simulink model "bh_2dof_NP_compare_lagr_vs_sm"  (R2017a)
settings: Solver=ode45  StartTime=0.0  StopTime=60  FixedStep=0.001  RelTol=1e-7  EnableMultiTasking=on
values from neighbouring files (symbols this model uses):
  theta1_0 = 0    [bh_SIMPARAMS_for_2dof_NP_Control_sim.m]
  theta1_dot_0 = 0    [bh_SIMPARAMS_for_2dof_NP_Control_sim.m]
  theta4_0 = 0    [bh_SIMPARAMS_for_2dof_NP_Control_sim.m]
  theta4_dot_0 = 0    [bh_SIMPARAMS_for_2dof_NP_Control_sim.m]
undefined symbols (not defined in the file or in its folder): b1_damp, b4_damp, g, Hz, L1x, L1y, L1z, mass1, mass4, Rturn, sigbuilder_block, X, Y, Z
libraries: simulink_extras x14, sm_lib x13, nesl_utility x9
settings Model: Creator=bhorton  LastModifiedBy=bhorton
settings SolverCC: ZeroCrossAlgorithm=Adaptive
settings OptimizationCC: LifeSpan=inf
settings DebuggingCC: SFUnexpectedBacktrackingDiag=warning  SFNoUnconditionalDefaultTransitionDiag=warning  SFExecutionAtInitializationDiag=none
settings GRTTargetCC: TargetLangStandard=C89/C90 (ANSI)
settings ConfigComp: CovMetricSettings=dw  CovHtmlReporting=on  CovSaveCumulativeToWorkspaceVar=on  CovSaveSingleToWorkspaceVar=on  CovExternalEMLEnable=off
settings SimscapeCC: SimscapeLogDataHistory=10000  SelectedTab=Simscape Multibody
settings ExplorerConfigSet: InternalSimMechanicsExplorerSettings="<ExplorerConfiguration><canonicalview>default</canonicalview><AnimationSetting><BasePlaybackSpeed>1.0</BasePlaybackSpeed><PlaybackSpeedFactor>1.0</PlaybackSpeedFactor></AnimationSetting><TilePanel><TileInfo><Tiles Columns=\"1\" Count=\"1\" Rows=\"1\"><Column Left=\"2\" Weight=\"1\"/><Column Left=\"820\" Weight=\"0.5006\"/><Row Top=\"2\" Weight=\"1\"/><Row Top=\"545\" Weight=\"0.5005\"/><Tile Height=\"1\" Width=\"1\" X=\"0\" Y=\"0\"/></Tiles></TileInfo><SceneInfo><SceneViewer><BGColor><R>0.60000002384185791</R><G>0.60000002384185791</G><B>0.60000002384185791</B></BGColor><Camera><DoPerspective>off</DoPerspective><Position><X>0.48444555295969882</X><Y>-0.15819555793399154</Y><Z>0.39694556248721286</Z></Position><Center><X>0.024999979464140232</X><Y>0.30125001556156705</Y><Z>-0.062500011008345735</Z></Center><Up><X>-0.40824829046386307</X><Y>0.40824829046386307</Y><Z>0.81649658092772615</Z></Up><ViewLimDist>1</ViewLimDist><YLim>0.27384785473346712</YLim><XLim>0.4148743716842227</XLim></Camera></SceneViewer></SceneInfo></TilePanel><MechEditorPanel><Cameras/><GfxPanelCameraMap/></MechEditorPanel></ExplorerConfiguration>"

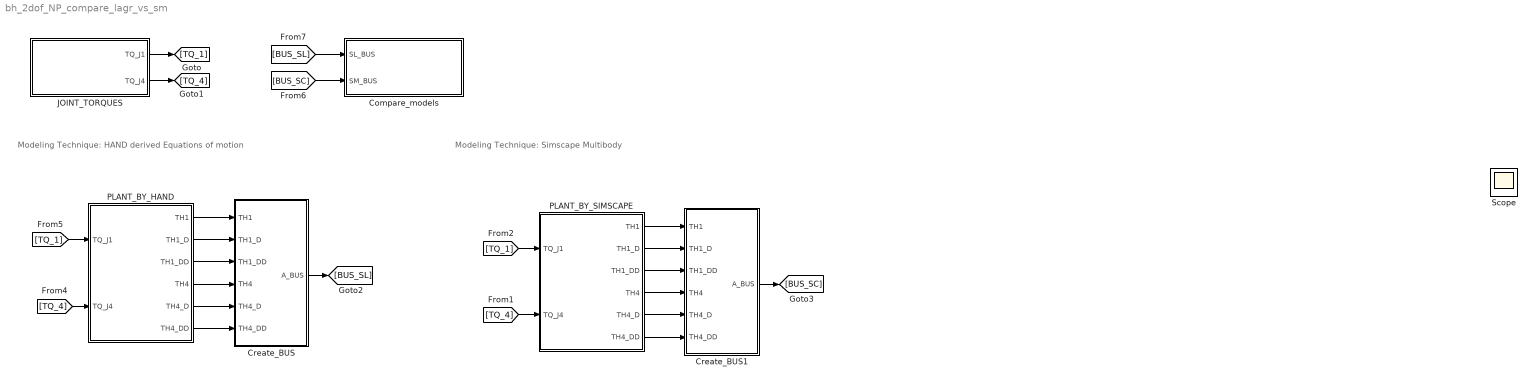
== system bh_2dof_NP_compare_lagr_vs_sm ==
  note: Modeling Technique: HAND derived Equations of motion
  note: Modeling Technique: Simscape Multibody
  Compare_models : Subsystem
  Create_BUS : Subsystem
  Create_BUS1 : Subsystem
  JOINT_TORQUES : Subsystem  Tag=STV Subsys  LoadFcn=sigbuilder_block('load');  StartFcn=sigbuilder_block('start');  StopFcn=sigbuilder_block('stop');  ClipboardFcn=sigbuilder_block('clipboard');  mask(Sigbuilder block){tuvar=[0:10]}
      mask help: Simulink:masks:SigbuilderBlock_MD
      mask init:
      | if ~strcmp(get_param(bdroot(gcbh),'SimulationStatus'),'stopped') tuvar = sigbuilder_block('maskInit'); end
      settings: CopyFcn=sigbuilder_block('copy');  DeleteFcn=sigbuilder_block('delete');  ModelCloseFcn=sigbuilder_block('modelClose');  PreSaveFcn=sigbuilder_block('preSave');  PauseFcn=sigbuilder_block('pause');  ContinueFcn=sigbuilder_block('continue');  NameChangeFcn=sigbuilder_block('namechange');  OpenFcn=sigbuilder_block('open',[6 30 1428 681.75 ]);  CloseFcn=sigbuilder_block('close');
      mask Display: plot(0, 0, 100, 100,[2, 2, 32, 32, 2], [68, 8, 8, 68, 68],[32, 2], [38, 38], [32, 19, 2],[53, 60, 44], [32, 17, 17, 2],[16, 16, 31, 31]);txt = getActiveGroup(gcbh);text(2, 100, txt,'verticalAlignment', 'top');
  PLANT_BY_HAND : Subsystem
  PLANT_BY_SIMSCAPE : Subsystem
  Scope : Scope
  wires:
  JOINT_TORQUES/1(TQ_J1) -> [TQ_1]
  JOINT_TORQUES/2(TQ_J4) -> [TQ_4]
  PLANT_BY_HAND/1(TH1) -> Create_BUS/1(TH1)
  PLANT_BY_HAND/2(TH1_D) -> Create_BUS/2(TH1_D)
  PLANT_BY_HAND/3(TH1_DD) -> Create_BUS/3(TH1_DD)
  PLANT_BY_HAND/4(TH4) -> Create_BUS/4(TH4)
  PLANT_BY_HAND/5(TH4_D) -> Create_BUS/5(TH4_D)
  PLANT_BY_HAND/6(TH4_DD) -> Create_BUS/6(TH4_DD)
  Create_BUS/1(A_BUS) -> [BUS_SL]
  PLANT_BY_SIMSCAPE/1(TH1) -> Create_BUS1/1(TH1)
  PLANT_BY_SIMSCAPE/2(TH1_D) -> Create_BUS1/2(TH1_D)
  PLANT_BY_SIMSCAPE/3(TH1_DD) -> Create_BUS1/3(TH1_DD)
  PLANT_BY_SIMSCAPE/4(TH4) -> Create_BUS1/4(TH4)
  PLANT_BY_SIMSCAPE/5(TH4_D) -> Create_BUS1/5(TH4_D)
  PLANT_BY_SIMSCAPE/6(TH4_DD) -> Create_BUS1/6(TH4_DD)
  Create_BUS1/1(A_BUS) -> [BUS_SC]
  [TQ_1] -> PLANT_BY_HAND/1("TQ_J1 ")
  [TQ_4] -> PLANT_BY_HAND/2(TQ_J4)
  [TQ_1] -> PLANT_BY_SIMSCAPE/1("TQ_J1 ")
  [TQ_4] -> PLANT_BY_SIMSCAPE/2(TQ_J4)
  [BUS_SL] -> Compare_models/1(SL_BUS)
  [BUS_SC] -> Compare_models/2(SM_BUS)

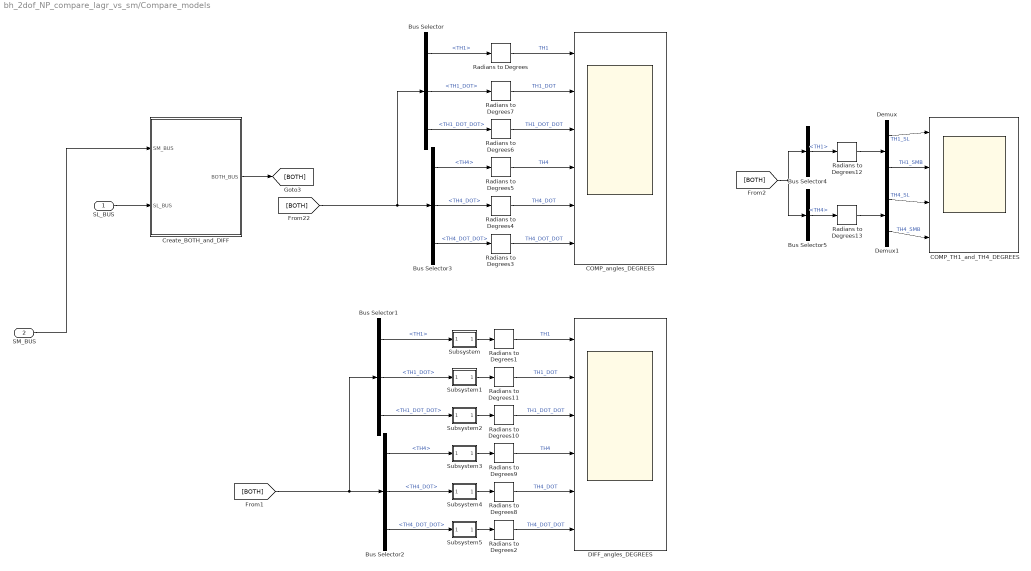
== system bh_2dof_NP_compare_lagr_vs_sm/Compare_models ==
  SL_BUS : Inport
  SM_BUS : Inport  Port=2
  Bus Selector : BusSelector  OutputSignals=TH1,TH1_DOT,TH1_DOT_DOT
  Bus Selector1 : BusSelector  OutputSignals=TH1,TH1_DOT,TH1_DOT_DOT
  Bus Selector2 : BusSelector  OutputSignals=TH4,TH4_DOT,TH4_DOT_DOT
  Bus Selector3 : BusSelector  OutputSignals=TH4,TH4_DOT,TH4_DOT_DOT
  Bus Selector4 : BusSelector  OutputSignals=TH1
  Bus Selector5 : BusSelector  OutputSignals=TH4
  COMP_TH1_and_TH4_DEGREES : Scope  NumInputPorts=4
  COMP_angles_DEGREES : Scope  NumInputPorts=6
  Create_BOTH_and_DIFF : Subsystem
  DIFF_angles_DEGREES : Scope  NumInputPorts=6
  Demux : Demux  Outputs=2
  Demux1 : Demux  Outputs=2
  Radians to Degrees{,1..13} (14 alike) : simulink_extras/Transformations/Radians to Degrees
  Subsystem : Subsystem
  Subsystem1 : Subsystem
  Subsystem2 : Subsystem
  Subsystem3 : Subsystem
  Subsystem4 : Subsystem
  Subsystem5 : Subsystem
  wires:
  SM_BUS/1 -> Create_BOTH_and_DIFF/1(SM_BUS)
  SL_BUS/1 -> Create_BOTH_and_DIFF/2(SL_BUS)
  Create_BOTH_and_DIFF/1(BOTH_BUS) -> [BOTH]
  Bus Selector/1 -> Radians to Degrees/1  "<TH1>"
  Bus Selector/2 -> Radians to Degrees7/1  "<TH1_DOT>"
  Bus Selector/3 -> Radians to Degrees6/1  "<TH1_DOT_DOT>"
  Bus Selector3/1 -> Radians to Degrees5/1  "<TH4>"
  Bus Selector3/2 -> Radians to Degrees4/1  "<TH4_DOT>"
  Bus Selector3/3 -> Radians to Degrees3/1  "<TH4_DOT_DOT>"
  [BOTH] -> Bus Selector/1, Bus Selector3/1
  Radians to Degrees/1 -> COMP_angles_DEGREES/1  "TH1"
  Radians to Degrees7/1 -> COMP_angles_DEGREES/2  "TH1_DOT"
  Radians to Degrees6/1 -> COMP_angles_DEGREES/3  "TH1_DOT_DOT"
  Radians to Degrees5/1 -> COMP_angles_DEGREES/4  "TH4"
  Radians to Degrees4/1 -> COMP_angles_DEGREES/5  "TH4_DOT"
  Radians to Degrees3/1 -> COMP_angles_DEGREES/6  "TH4_DOT_DOT"
  Bus Selector1/1 -> Subsystem/1(In1)  "<TH1>"
  Bus Selector1/2 -> Subsystem1/1(In1)  "<TH1_DOT>"
  Bus Selector1/3 -> Subsystem2/1(In1)  "<TH1_DOT_DOT>"
  Bus Selector2/1 -> Subsystem3/1(In1)  "<TH4>"
  Bus Selector2/2 -> Subsystem4/1(In1)  "<TH4_DOT>"
  Bus Selector2/3 -> Subsystem5/1(In1)  "<TH4_DOT_DOT>"
  [BOTH] -> Bus Selector1/1, Bus Selector2/1
  Radians to Degrees1/1 -> DIFF_angles_DEGREES/1  "TH1"
  Radians to Degrees11/1 -> DIFF_angles_DEGREES/2  "TH1_DOT"
  Radians to Degrees10/1 -> DIFF_angles_DEGREES/3  "TH1_DOT_DOT"
  Radians to Degrees9/1 -> DIFF_angles_DEGREES/4  "TH4"
  Radians to Degrees8/1 -> DIFF_angles_DEGREES/5  "TH4_DOT"
  Radians to Degrees2/1 -> DIFF_angles_DEGREES/6  "TH4_DOT_DOT"
  Subsystem/1(diff) -> Radians to Degrees1/1
  Subsystem5/1(diff) -> Radians to Degrees2/1
  Subsystem4/1(diff) -> Radians to Degrees8/1
  Subsystem3/1(diff) -> Radians to Degrees9/1
  Subsystem2/1(diff) -> Radians to Degrees10/1
  Subsystem1/1(diff) -> Radians to Degrees11/1
  [BOTH] -> Bus Selector4/1, Bus Selector5/1
  Bus Selector5/1 -> Radians to Degrees13/1  "<TH4>"
  Bus Selector4/1 -> Radians to Degrees12/1  "<TH1>"
  Radians to Degrees12/1 -> Demux/1
  Radians to Degrees13/1 -> Demux1/1
  Demux1/1 -> COMP_TH1_and_TH4_DEGREES/3  "TH4_SL"
  Demux1/2 -> COMP_TH1_and_TH4_DEGREES/4  "TH4_SMB"
  Demux/1 -> COMP_TH1_and_TH4_DEGREES/1  "TH1_SL"
  Demux/2 -> COMP_TH1_and_TH4_DEGREES/2  "TH1_SMB"

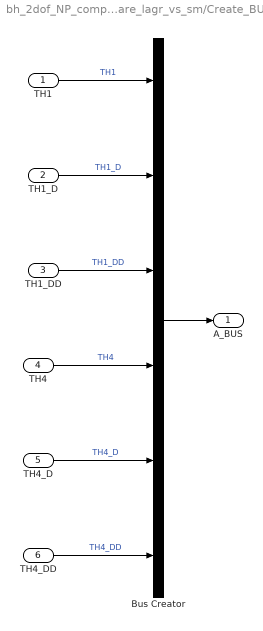
== system bh_2dof_NP_compare_lagr_vs_sm/Create_BUS ==
  TH1 : Inport
  TH1_D : Inport  Port=2
  TH1_DD : Inport  Port=3
  TH4 : Inport  Port=4
  TH4_D : Inport  Port=5
  TH4_DD : Inport  Port=6
  Bus Creator : BusCreator  Inputs=6
  A_BUS : Outport
  wires:
  TH1_DD/1 -> Bus Creator/3  "TH1_DD"
  TH1_D/1 -> Bus Creator/2  "TH1_D"
  TH1/1 -> Bus Creator/1  "TH1"
  Bus Creator/1 -> A_BUS/1
  TH4_DD/1 -> Bus Creator/6  "TH4_DD"
  TH4_D/1 -> Bus Creator/5  "TH4_D"
  TH4/1 -> Bus Creator/4  "TH4"

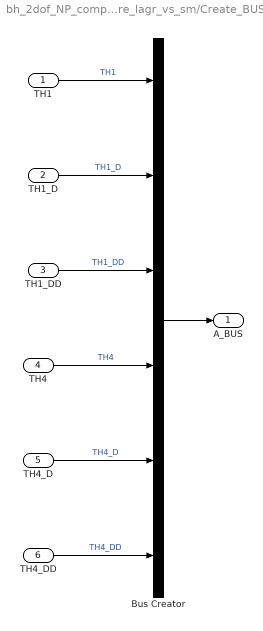
== system bh_2dof_NP_compare_lagr_vs_sm/Create_BUS1 ==
  TH1 : Inport
  TH1_D : Inport  Port=2
  TH1_DD : Inport  Port=3
  TH4 : Inport  Port=4
  TH4_D : Inport  Port=5
  TH4_DD : Inport  Port=6
  Bus Creator : BusCreator  Inputs=6
  A_BUS : Outport
  wires:
  TH1_DD/1 -> Bus Creator/3  "TH1_DD"
  TH1_D/1 -> Bus Creator/2  "TH1_D"
  TH1/1 -> Bus Creator/1  "TH1"
  Bus Creator/1 -> A_BUS/1
  TH4_DD/1 -> Bus Creator/6  "TH4_DD"
  TH4_D/1 -> Bus Creator/5  "TH4_D"
  TH4/1 -> Bus Creator/4  "TH4"

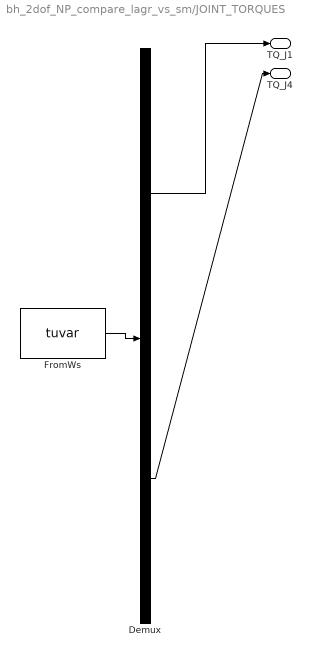
== system bh_2dof_NP_compare_lagr_vs_sm/JOINT_TORQUES ==
  Demux : Demux  Tag=STV Demux  Outputs=2
  FromWs : FromWorkspace  Tag=STV FromWs  VariableName=tuvar  SampleTime=0
      SigBuilderData=|
      | common.afterFinalStr = 'Extrapolate'
      | common.sampleTime = 0
      | dataSet(1).timeRange = [0 60]
      | dataSet(1).name = 'PULSES_SMALL'
      | dataSet(2).timeRange = [0 1000]
      | dataSet(2).name = 'ZERO'
      | dataSet(3).timeRange = [0 1000]
      | dataSet(3).name = 'PULSES_BIG'
      | dataSet(4).timeRange = [0 70]
      | dataSet(4).name = 'Motor_TQs'
      | sbobj.Groups(1).Name = 'PULSES_SMALL'
      | sbobj.Groups(1).Signals(1).Name = 'TQ_J1'
      | sbobj.Groups(1).Signals(1).XData = [0 20 20 35 35 60]
      | sbobj.Groups(1).Signals(1).YData = [0 0 0.348 0.348 0 0]
      | sbobj.Groups(1).Signals(2).Name = 'TQ_J4'
      | sbobj.Groups(1).Signals(2).XData = [0 25 25 40 40 60]
      | sbobj.Groups(1).Signals(2).YData = [0 0 0.1 0.1 0 0]
      | sbobj.Groups(1).TimeRange = [0 60]
      | sbobj.Groups(2).Name = 'ZERO'
      | sbobj.Groups(2).Signals(1).Name = 'TQ_J1'
      | sbobj.Groups(2).Signals(1).XData = [0 600 612 1000]
      | sbobj.Groups(2).Signals(1).YData = [0 0 0 0]
      | sbobj.Groups(2).Signals(2).Name = 'TQ_J4'
      | sbobj.Groups(2).Signals(2).XData = [0 888 902 1000]
      | sbobj.Groups(2).Signals(2).YData = [0 0 0 0]
      | sbobj.Groups(2).TimeRange = [0 1000]
      | sbobj.Groups(3).Name = 'PULSES_BIG'
      | sbobj.Groups(3).Signals(1).Name = 'TQ_J1'
      | sbobj.Groups(3).Signals(1).XData = [0 600 600 692 692 1000]
      | sbobj.Groups(3).Signals(1).YData = [0 0 0.1 0.1 0 0]
      | sbobj.Groups(3).Signals(2).Name = 'TQ_J4'
      | sbobj.Groups(3).Signals(2).XData = [0 500 500 840 840 1000]
      | sbobj.Groups(3).Signals(2).YData = [0 0 0.016 0.016 0 0]
      | sbobj.Groups(3).TimeRange = [0 1000]
      | sbobj.Groups(4).Name = 'Motor_TQs'
      | sbobj.Groups(4).Signals(1).Name = 'TQ_J1'
      | sbobj.Groups(4).Signals(1).XData = [0 2.16837330161e-09 1.30102398096e-08 3.17295560441e-08 5.69304221095e-08 8.75590864979e-08 1.2292243537e-07 1.62530861971e-07 2.06018177113e-07 2.53098604874e-07 3.03541856444e-07 3.57157698409e-07 ... (13166 elements, 1x13166)]
      | sbobj.Groups(4).Signals(1).YData = [-3.69730691656 -3.69730688652 -3.69730673619 -3.69730647615 -3.69730612512 -3.69730569704 -3.6973052008 -3.69730464247 -3.69730402639 -3.69730335581 -3.69730263318 -3.69730186041 ... (13166 elements, 1x13166)]
      | sbobj.Groups(4).Signals(2).Name = 'TQ_J4'
      | sbobj.Groups(4).Signals(2).XData = [0 2.16837330161e-09 1.30102398096e-08 3.17295560441e-08 5.69304221095e-08 8.75590864979e-08 1.2292243537e-07 1.62530861971e-07 2.06018177113e-07 2.53098604874e-07 3.03541856444e-07 3.57157698409e-07 ... (13166 elements, 1x13166)]
      | sbobj.Groups(4).Signals(2).YData = [-2.92455799646 -2.92455799836 -2.92455800761 -2.92455802275 -2.92455804143 -2.92455806151 -2.92455808113 -2.92455809856 -2.92455811219 -2.92455812047 -2.92455812186 -2.9245581149 ... (13166 elements, 1x13166)]
      | sbobj.Groups(4).TimeRange = [0 70]
  TQ_J1 : Outport  Tag=STV Outport
  TQ_J4 : Outport  Tag=STV Outport  Port=2
  wires:
  Demux/1 -> TQ_J1/1
  FromWs/1 -> Demux/1
  Demux/2 -> TQ_J4/1

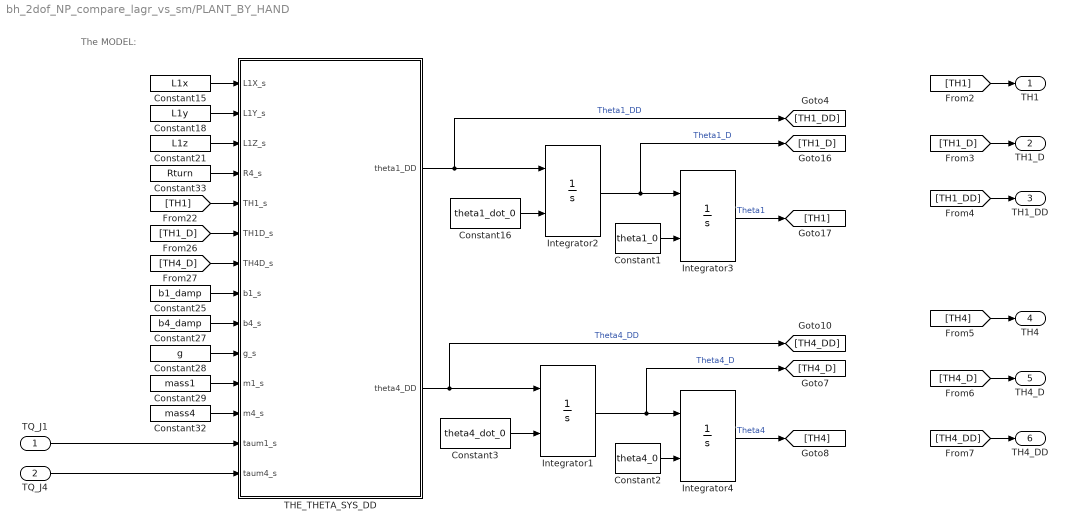
== system bh_2dof_NP_compare_lagr_vs_sm/PLANT_BY_HAND ==
  note: The MODEL:
  "TQ_J1 " : Inport
  TQ_J4 : Inport  Port=2
  Constant1 : Constant  Value=theta1_0
  Constant15 : Constant  Value=L1x
  Constant16 : Constant  Value=theta1_dot_0
  Constant18 : Constant  Value=L1y
  Constant2 : Constant  Value=theta4_0
  Constant21 : Constant  Value=L1z
  Constant25 : Constant  Value=b1_damp
  Constant27 : Constant  Value=b4_damp
  Constant28 : Constant  Value=g
  Constant29 : Constant  Value=mass1
  Constant3 : Constant  Value=theta4_dot_0
  Constant32 : Constant  Value=mass4
  Constant33 : Constant  Value=Rturn
  Integrator{1..4} (4 alike) : Integrator  InitialConditionSource=external
  THE_THETA_SYS_DD : MATLAB Function  TreatAsAtomicUnit=on
  TH1 : Outport
  TH1_D : Outport  Port=2
  TH1_DD : Outport  Port=3
  TH4 : Outport  Port=4
  TH4_D : Outport  Port=5
  TH4_DD : Outport  Port=6
  wires:
  [TH4_D] -> TH4_D/1
  Constant16/1 -> Integrator2/2
  Integrator2/1 -> [TH1_D], Integrator3/1  "Theta1_D"
  TQ_J4/1 -> THE_THETA_SYS_DD/14(taum4_s)
  Integrator4/1 -> [TH4]  "Theta4"
  [TH4_D] -> THE_THETA_SYS_DD/7(TH4D_s)
  [TH1] -> THE_THETA_SYS_DD/5(TH1_s)
  [TH1_DD] -> TH1_DD/1
  Constant29/1 -> THE_THETA_SYS_DD/11(m1_s)
  Constant33/1 -> THE_THETA_SYS_DD/4(R4_s)
  THE_THETA_SYS_DD/1(theta1_DD) -> [TH1_DD], Integrator2/1  "Theta1_DD"
  Integrator3/1 -> [TH1]  "Theta1"
  Constant18/1 -> THE_THETA_SYS_DD/2(L1Y_s)
  THE_THETA_SYS_DD/2(theta4_DD) -> Integrator1/1, [TH4_DD]  "Theta4_DD"
  Constant2/1 -> Integrator4/2
  "TQ_J1 "/1 -> THE_THETA_SYS_DD/13(taum1_s)
  [TH1] -> TH1/1
  Constant1/1 -> Integrator3/2
  Constant27/1 -> THE_THETA_SYS_DD/9(b4_s)
  [TH1_D] -> TH1_D/1
  Constant32/1 -> THE_THETA_SYS_DD/12(m4_s)
  [TH4_DD] -> TH4_DD/1
  Constant3/1 -> Integrator1/2
  Constant25/1 -> THE_THETA_SYS_DD/8(b1_s)
  [TH4] -> TH4/1
  Constant15/1 -> THE_THETA_SYS_DD/1(L1X_s)
  Constant21/1 -> THE_THETA_SYS_DD/3(L1Z_s)
  [TH1_D] -> THE_THETA_SYS_DD/6(TH1D_s)
  Integrator1/1 -> [TH4_D], Integrator4/1  "Theta4_D"
  Constant28/1 -> THE_THETA_SYS_DD/10(g_s)

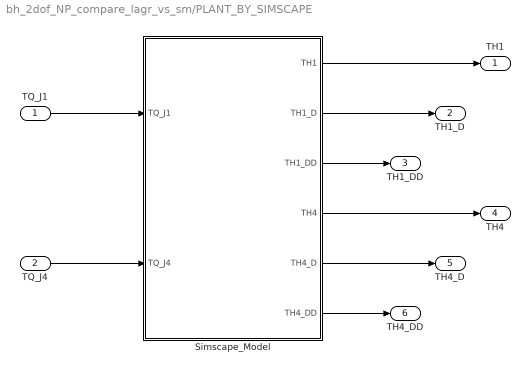
== system bh_2dof_NP_compare_lagr_vs_sm/PLANT_BY_SIMSCAPE ==
  "TQ_J1 " : Inport
  TQ_J4 : Inport  Port=2
  Simscape_Model : Subsystem  VariantControl=Variant1
  TH1 : Outport
  TH1_D : Outport  Port=2
  TH1_DD : Outport  Port=3
  TH4 : Outport  Port=4
  TH4_D : Outport  Port=5
  TH4_DD : Outport  Port=6
  wires:
  TQ_J4/1 -> Simscape_Model/2(TQ_J4)
  "TQ_J1 "/1 -> Simscape_Model/1("TQ_J1 ")
  Simscape_Model/1(TH1) -> TH1/1
  Simscape_Model/2(TH1_D) -> TH1_D/1
  Simscape_Model/3(TH1_DD) -> TH1_DD/1
  Simscape_Model/6(TH4_DD) -> TH4_DD/1
  Simscape_Model/5(TH4_D) -> TH4_D/1
  Simscape_Model/4(TH4) -> TH4/1

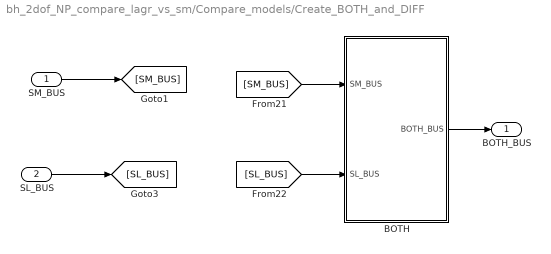
== system bh_2dof_NP_compare_lagr_vs_sm/Compare_models/Create_BOTH_and_DIFF ==
  SM_BUS : Inport
  SL_BUS : Inport  Port=2
  BOTH : Subsystem
  BOTH_BUS : Outport
  wires:
  SL_BUS/1 -> [SL_BUS]
  SM_BUS/1 -> [SM_BUS]
  [SM_BUS] -> BOTH/1(SM_BUS)
  [SL_BUS] -> BOTH/2(SL_BUS)
  BOTH/1(BOTH_BUS) -> BOTH_BUS/1

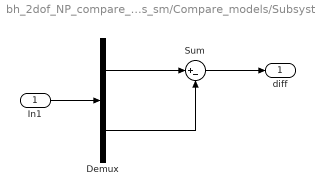
== system bh_2dof_NP_compare_lagr_vs_sm/Compare_models/Subsystem ==
  In1 : Inport
  Demux : Demux  Outputs=2
  Sum : Sum  Inputs=|+-
  diff : Outport
  wires:
  In1/1 -> Demux/1
  Demux/1 -> Sum/1
  Demux/2 -> Sum/2
  Sum/1 -> diff/1

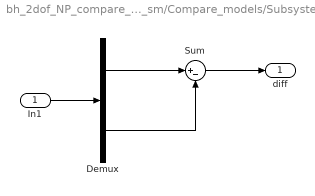
== system bh_2dof_NP_compare_lagr_vs_sm/Compare_models/Subsystem1 ==
  In1 : Inport
  Demux : Demux  Outputs=2
  Sum : Sum  Inputs=|+-
  diff : Outport
  wires:
  In1/1 -> Demux/1
  Demux/1 -> Sum/1
  Demux/2 -> Sum/2
  Sum/1 -> diff/1

== system bh_2dof_NP_compare_lagr_vs_sm/Compare_models/Subsystem2 ==
  In1 : Inport
  Demux : Demux  Outputs=2
  Sum : Sum  Inputs=|+-
  diff : Outport
  wires:
  In1/1 -> Demux/1
  Demux/1 -> Sum/1
  Demux/2 -> Sum/2
  Sum/1 -> diff/1

== system bh_2dof_NP_compare_lagr_vs_sm/Compare_models/Subsystem3 ==
  In1 : Inport
  Demux : Demux  Outputs=2
  Sum : Sum  Inputs=|+-
  diff : Outport
  wires:
  In1/1 -> Demux/1
  Demux/1 -> Sum/1
  Demux/2 -> Sum/2
  Sum/1 -> diff/1

== system bh_2dof_NP_compare_lagr_vs_sm/Compare_models/Subsystem4 ==
  In1 : Inport
  Demux : Demux  Outputs=2
  Sum : Sum  Inputs=|+-
  diff : Outport
  wires:
  In1/1 -> Demux/1
  Demux/1 -> Sum/1
  Demux/2 -> Sum/2
  Sum/1 -> diff/1

== system bh_2dof_NP_compare_lagr_vs_sm/Compare_models/Subsystem5 ==
  In1 : Inport
  Demux : Demux  Outputs=2
  Sum : Sum  Inputs=|+-
  diff : Outport
  wires:
  In1/1 -> Demux/1
  Demux/1 -> Sum/1
  Demux/2 -> Sum/2
  Sum/1 -> diff/1

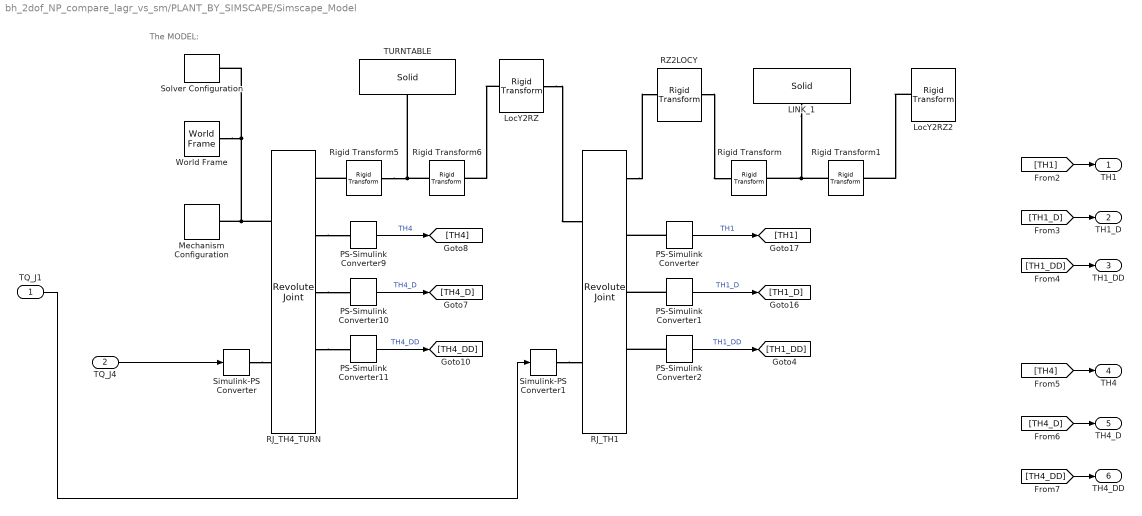
== system bh_2dof_NP_compare_lagr_vs_sm/PLANT_BY_SIMSCAPE/Simscape_Model ==
  note: The MODEL:
  "TQ_J1 " : Inport
  TQ_J4 : Inport  Port=2
  LINK_1 : sm_lib/Body Elements/Solid  InertiaType=CalculateFromGeometry  Mass=1  MassUnits=kg  CenterOfMass=[0 0 0]  CenterOfMassUnits=m  MomentsOfInertia=[1 1 1]  MomentsOfInertiaUnits=kg*m^2  ProductsOfInertia=[0 0 0]  ProductsOfInertiaUnits=kg*m^2  DensityBased=on  Density=density  DensityUnits=kg/(m^3)  DoExposeReferenceFrame=on  SerializedFrames=<Frames/>  GraphicType=FromGeometry  MarkerShape=Sphere  MarkerSize=10  GraphicVisPropType=SimpleVisualProperties  GraphicDiffuseColor=[0.2 0.2 1.0]  GraphicSpecularColor=[0.5 0.5 0.5 1.0]  GraphicAmbientColor=[0.15 0.15 0.15 1.0]  GraphicEmissiveColor=[0.0 0.0 0.0 1.0]  GraphicShininess=75  GraphicOpacity=1.0  GeometryShape=Brick  RectangleSize=[1 1]  RectangleSizeUnits=m  BrickDimensions=[L1x, L1y, L1z ]  BrickDimensionUnits=m  CylinderRadius=1  CylinderRadiusUnits=m  CylinderLength=1  CylinderLengthUnits=m  SphereRadius=1  SphereRadiusUnits=m  EllipsoidRadii=[1 1 1]  EllipsoidRadiiUnits=m  ExtrusionCrossSection=[1 1; -1 1; -1 -1; 1 -1]  ExtrusionCrossSectionUnits=m  ExtrusionLength=1  ExtrusionLengthUnits=m  PolygonNumSides=3  PolygonOuterRadius=1  PolygonOuterRadiusUnits=m  ExtGeomFileType=STEP  ExtGeomFileUnits=m  RevolutionCrossSection=[1 1; 1 -1; 2 -1; 2 1]  RevolutionCrossSectionUnits=m  RevolutionExtent=Full  RevolutionAngle=180  RevolutionAngleUnits=deg
  LocY2RZ : sm_lib/Frames and Transforms/Rigid Transform  TranslationMethod=None  TranslationStandardOffset=Hz/2  TranslationLengthUnit=m  TranslationStandardAxis=+Z  TranslationCartesianOffset=[0 0 0]  TranslationROffset=0  TranslationROffsetUnits=m  TranslationZOffset=0  TranslationZOffsetUnits=m  TranslationThetaOffset=0  TranslationThetaOffsetUnits=deg  RotationMethod=AlignedAxes  RotationAngleUnits=deg  RotationStandardAxis=+Z  RotationAngle=0.0  RotationArbitraryAxis=[0 0 1]  FollAlignAxisA=+X  BaseAlignAxisA=+Y  FollAlignAxisB=+Y  BaseAlignAxisB=+Z  RotationSequenceAxes=FollowerAxes  RotationSequence=XYX  RotationSequenceAngles=[0 0 0]  RotationSequenceAnglesUnits=deg  RotationMatrix=[1 0 0; 0 1 0; 0 0 1]
  LocY2RZ2 : sm_lib/Frames and Transforms/Rigid Transform  TranslationMethod=None  TranslationStandardOffset=Hz/2  TranslationLengthUnit=m  TranslationStandardAxis=+Z  TranslationCartesianOffset=[0 0 0]  TranslationROffset=0  TranslationROffsetUnits=m  TranslationZOffset=0  TranslationZOffsetUnits=m  TranslationThetaOffset=0  TranslationThetaOffsetUnits=deg  RotationMethod=AlignedAxes  RotationAngleUnits=deg  RotationStandardAxis=+Z  RotationAngle=0.0  RotationArbitraryAxis=[0 0 1]  FollAlignAxisA=+X  BaseAlignAxisA=+Y  FollAlignAxisB=+Y  BaseAlignAxisB=+Z  RotationSequenceAxes=FollowerAxes  RotationSequence=XYX  RotationSequenceAngles=[0 0 0]  RotationSequenceAnglesUnits=deg  RotationMatrix=[1 0 0; 0 1 0; 0 0 1]
  Mechanism Configuration : sm_lib/Utilities/Mechanism Configuration  UniformGravity=Constant  GravityVector=[0 0 -g ]  GravityUnits=m/s^2  LinearizationDelta=1e-4
  PS-Simulink Converter : nesl_utility/PS-Simulink Converter  PhysicalDomain=network_engine_domain  SubClassName=ps_output  LeftPortType=input  RightPortType=output  PseudoPeriodic=off  Frequencies=[]  Unit=rad  AffineConversion=off
  PS-Simulink Converter1 : nesl_utility/PS-Simulink Converter  PhysicalDomain=network_engine_domain  SubClassName=ps_output  LeftPortType=input  RightPortType=output  PseudoPeriodic=off  Frequencies=[]  Unit=rad/s  AffineConversion=off
  PS-Simulink Converter10 : nesl_utility/PS-Simulink Converter  PhysicalDomain=network_engine_domain  SubClassName=ps_output  LeftPortType=input  RightPortType=output  PseudoPeriodic=off  Frequencies=[]  Unit=rad/s  AffineConversion=off
  PS-Simulink Converter11 : nesl_utility/PS-Simulink Converter  PhysicalDomain=network_engine_domain  SubClassName=ps_output  LeftPortType=input  RightPortType=output  PseudoPeriodic=off  Frequencies=[]  Unit=rad/s^2  AffineConversion=off
  PS-Simulink Converter2 : nesl_utility/PS-Simulink Converter  PhysicalDomain=network_engine_domain  SubClassName=ps_output  LeftPortType=input  RightPortType=output  PseudoPeriodic=off  Frequencies=[]  Unit=rad/s^2  AffineConversion=off
  PS-Simulink Converter9 : nesl_utility/PS-Simulink Converter  PhysicalDomain=network_engine_domain  SubClassName=ps_output  LeftPortType=input  RightPortType=output  PseudoPeriodic=off  Frequencies=[]  Unit=rad  AffineConversion=off
  RJ_TH1 : sm_lib/Joints/Revolute Joint  SenseConstraintForce=on  SenseConstraintForceX=off  SenseConstraintForceY=off  SenseConstraintForceZ=off  SenseConstraintTorque=off  SenseConstraintTorqueX=off  SenseConstraintTorqueY=off  SenseConstraintTorqueZ=off  SenseTotalForce=off  SenseTotalForceX=off  SenseTotalForceY=off  SenseTotalForceZ=off  SenseTotalTorque=off  SenseTotalTorqueX=off  SenseTotalTorqueY=off  SenseTotalTorqueZ=off  CompositeWrenchDir=BaseOnFollower  CompositeWrenchFrame=BaseFrame  EquilibriumPosition=0  EquilibriumPositionUnits=deg  SpringStiffness=0  SpringStiffnessUnits=N*m/deg  DampingCoefficient=b1_damp  DampingCoefficientUnits=N*m/(rad/s)  TorqueActuationMode=InputTorque  MotionActuationMode=ComputedMotion  SensePosition=on  SenseVelocity=on  SenseAcceleration=on  SenseTorqueForce=off  PositionTargetSpecify=on  PositionTargetPriority=Low  PositionTargetValue=theta1_0  PositionTargetValueUnits=rad  VelocityTargetSpecify=on  VelocityTargetPriority=High  VelocityTargetValue=theta1_dot_0  VelocityTargetValueUnits=rad/s
      settings: AttributesFormatString=|
      | %<DampingCoefficient>
      | %<PositionTargetValue>
      | %<VelocityTargetValue>
  RJ_TH4_TURN : sm_lib/Joints/Revolute Joint  SenseConstraintForce=on  SenseConstraintForceX=off  SenseConstraintForceY=off  SenseConstraintForceZ=off  SenseConstraintTorque=off  SenseConstraintTorqueX=off  SenseConstraintTorqueY=off  SenseConstraintTorqueZ=off  SenseTotalForce=off  SenseTotalForceX=off  SenseTotalForceY=off  SenseTotalForceZ=off  SenseTotalTorque=off  SenseTotalTorqueX=off  SenseTotalTorqueY=off  SenseTotalTorqueZ=off  CompositeWrenchDir=BaseOnFollower  CompositeWrenchFrame=BaseFrame  EquilibriumPosition=0  EquilibriumPositionUnits=deg  SpringStiffness=0  SpringStiffnessUnits=N*m/deg  DampingCoefficient=b4_damp  DampingCoefficientUnits=N*m/(rad/s)  TorqueActuationMode=InputTorque  MotionActuationMode=ComputedMotion  SensePosition=on  SenseVelocity=on  SenseAcceleration=on  SenseTorqueForce=off  PositionTargetSpecify=on  PositionTargetPriority=Low  PositionTargetValue=theta4_0  PositionTargetValueUnits=rad  VelocityTargetSpecify=on  VelocityTargetPriority=High  VelocityTargetValue=theta4_dot_0  VelocityTargetValueUnits=rad/s
      settings: AttributesFormatString=|
      | %<DampingCoefficient>
      | %<PositionTargetValue>
      | %<VelocityTargetValue>
  RZ2LOCY : sm_lib/Frames and Transforms/Rigid Transform  TranslationMethod=None  TranslationStandardOffset=Hz/2  TranslationLengthUnit=m  TranslationStandardAxis=+Z  TranslationCartesianOffset=[0 0 0]  TranslationROffset=0  TranslationROffsetUnits=m  TranslationZOffset=0  TranslationZOffsetUnits=m  TranslationThetaOffset=0  TranslationThetaOffsetUnits=deg  RotationMethod=AlignedAxes  RotationAngleUnits=deg  RotationStandardAxis=+Z  RotationAngle=0.0  RotationArbitraryAxis=[0 0 1]  FollAlignAxisA=+Y  BaseAlignAxisA=+X  FollAlignAxisB=+X  BaseAlignAxisB=+Z  RotationSequenceAxes=FollowerAxes  RotationSequence=XYX  RotationSequenceAngles=[0 0 0]  RotationSequenceAnglesUnits=deg  RotationMatrix=[1 0 0; 0 1 0; 0 0 1]
  Rigid Transform : sm_lib/Frames and Transforms/Rigid Transform  TranslationMethod=StandardAxis  TranslationStandardOffset=L1y/2  TranslationLengthUnit=m  TranslationStandardAxis=+Y  TranslationCartesianOffset=[0 0 0]  TranslationROffset=0  TranslationROffsetUnits=m  TranslationZOffset=0  TranslationZOffsetUnits=m  TranslationThetaOffset=0  TranslationThetaOffsetUnits=deg  RotationMethod=None  RotationAngleUnits=deg  RotationStandardAxis=+Z  RotationAngle=0.0  RotationArbitraryAxis=[0 0 1]  FollAlignAxisA=+X  BaseAlignAxisA=+Y  FollAlignAxisB=+Y  BaseAlignAxisB=+Z  RotationSequenceAxes=FollowerAxes  RotationSequence=XYX  RotationSequenceAngles=[0 0 0]  RotationSequenceAnglesUnits=deg  RotationMatrix=[1 0 0; 0 1 0; 0 0 1]
  Rigid Transform1 : sm_lib/Frames and Transforms/Rigid Transform  TranslationMethod=StandardAxis  TranslationStandardOffset=L1y/2  TranslationLengthUnit=m  TranslationStandardAxis=+Y  TranslationCartesianOffset=[0 0 0]  TranslationROffset=0  TranslationROffsetUnits=m  TranslationZOffset=0  TranslationZOffsetUnits=m  TranslationThetaOffset=0  TranslationThetaOffsetUnits=deg  RotationMethod=None  RotationAngleUnits=deg  RotationStandardAxis=+Z  RotationAngle=0.0  RotationArbitraryAxis=[0 0 1]  FollAlignAxisA=+X  BaseAlignAxisA=+Y  FollAlignAxisB=+Y  BaseAlignAxisB=+Z  RotationSequenceAxes=FollowerAxes  RotationSequence=XYX  RotationSequenceAngles=[0 0 0]  RotationSequenceAnglesUnits=deg  RotationMatrix=[1 0 0; 0 1 0; 0 0 1]
  Rigid Transform5 : sm_lib/Frames and Transforms/Rigid Transform  TranslationMethod=StandardAxis  TranslationStandardOffset=Hz/2  TranslationLengthUnit=m  TranslationStandardAxis=-Z  TranslationCartesianOffset=[0 0 0]  TranslationROffset=0  TranslationROffsetUnits=m  TranslationZOffset=0  TranslationZOffsetUnits=m  TranslationThetaOffset=0  TranslationThetaOffsetUnits=deg  RotationMethod=None  RotationAngleUnits=deg  RotationStandardAxis=+Z  RotationAngle=0.0  RotationArbitraryAxis=[0 0 1]  FollAlignAxisA=+X  BaseAlignAxisA=+Y  FollAlignAxisB=+Y  BaseAlignAxisB=+Z  RotationSequenceAxes=FollowerAxes  RotationSequence=XYX  RotationSequenceAngles=[0 0 0]  RotationSequenceAnglesUnits=deg  RotationMatrix=[1 0 0; 0 1 0; 0 0 1]
  Rigid Transform6 : sm_lib/Frames and Transforms/Rigid Transform  TranslationMethod=StandardAxis  TranslationStandardOffset=Hz/2  TranslationLengthUnit=m  TranslationStandardAxis=+Z  TranslationCartesianOffset=[0 0 0]  TranslationROffset=0  TranslationROffsetUnits=m  TranslationZOffset=0  TranslationZOffsetUnits=m  TranslationThetaOffset=0  TranslationThetaOffsetUnits=deg  RotationMethod=None  RotationAngleUnits=deg  RotationStandardAxis=+Z  RotationAngle=0.0  RotationArbitraryAxis=[0 0 1]  FollAlignAxisA=+X  BaseAlignAxisA=+Y  FollAlignAxisB=+Y  BaseAlignAxisB=+Z  RotationSequenceAxes=FollowerAxes  RotationSequence=XYX  RotationSequenceAngles=[0 0 0]  RotationSequenceAnglesUnits=deg  RotationMatrix=[1 0 0; 0 1 0; 0 0 1]
  Simulink-PS Converter : nesl_utility/Simulink-PS Converter  PhysicalDomain=network_engine_domain  SubClassName=ps_input  LeftPortType=input  RightPortType=output  PseudoPeriodic=off  Frequencies=[]  NoiseDistribution=none  NoiseParameters=[]  Unit=N*m  AffineConversion=off  FilteringAndDerivatives=zero  SimscapeFilterOrder=1  InputFilterTimeConstant=0.001  UdotUserProvided=1
  Simulink-PS Converter1 : nesl_utility/Simulink-PS Converter  PhysicalDomain=network_engine_domain  SubClassName=ps_input  LeftPortType=input  RightPortType=output  PseudoPeriodic=off  Frequencies=[]  NoiseDistribution=none  NoiseParameters=[]  Unit=N*m  AffineConversion=off  FilteringAndDerivatives=zero  SimscapeFilterOrder=1  InputFilterTimeConstant=0.001  UdotUserProvided=1
  Solver Configuration : nesl_utility/Solver Configuration  PhysicalDomain=network_engine_domain  SubClassName=solver  LeftPortType=input  RightPortType=generic  Accelerate=off  Tones=[]  Harmonics=[]  SimulateNoise=off  Profile=off  UseLocalSampling=off  EnableSwitchedLinearOptims=on  FrequencyDomain=off  UseCCode=off  RelTol=0.001  AbsTol=1e-06  MinStep=1e-09  ToWorkspace=off  RevertToSquareIcSolve=off  NumHomotopyIterations=100  PhasorMode=off  PhasorModeNumHarmonics=1  OverrideAbsTol=off  DoDC=off  ResidualTolerance=1e-09  UseLocalSolver=off  LocalSolverChoice=NE_TRAPEZOIDAL_ADVANCER  LocalSolverSampleTime=0.01  DoFixedCost=off  MaxNonlinIter=3  MaxModeIter=2  LinearAlgebra=Sparse  DelaysMemoryBudget=1024  AutomaticFiltering=off  FilteringTimeConstant=0.001
  TURNTABLE : sm_lib/Body Elements/Solid  InertiaType=CalculateFromGeometry  Mass=1  MassUnits=kg  CenterOfMass=[0 0 0]  CenterOfMassUnits=m  MomentsOfInertia=[1 1 1]  MomentsOfInertiaUnits=kg*m^2  ProductsOfInertia=[0 0 0]  ProductsOfInertiaUnits=kg*m^2  DensityBased=on  Density=density  DensityUnits=kg/(m^3)  DoExposeReferenceFrame=on  SerializedFrames=<Frames/>  GraphicType=FromGeometry  MarkerShape=Sphere  MarkerSize=10  GraphicVisPropType=SimpleVisualProperties  GraphicDiffuseColor=[1.0 1.0 0.2]  GraphicSpecularColor=[0.5 0.5 0.5 1.0]  GraphicAmbientColor=[0.15 0.15 0.15 1.0]  GraphicEmissiveColor=[0.0 0.0 0.0 1.0]  GraphicShininess=75  GraphicOpacity=1.0  GeometryShape=Cylinder  RectangleSize=[1 1]  RectangleSizeUnits=m  BrickDimensions=[1 1 1]  BrickDimensionUnits=m  CylinderRadius=Rturn  CylinderRadiusUnits=m  CylinderLength=Hz  CylinderLengthUnits=m  SphereRadius=1  SphereRadiusUnits=m  EllipsoidRadii=[1 1 1]  EllipsoidRadiiUnits=m  ExtrusionCrossSection=[1 1; -1 1; -1 -1; 1 -1]  ExtrusionCrossSectionUnits=m  ExtrusionLength=1  ExtrusionLengthUnits=m  PolygonNumSides=3  PolygonOuterRadius=1  PolygonOuterRadiusUnits=m  ExtGeomFileType=STEP  ExtGeomFileUnits=m  RevolutionCrossSection=[1 1; 1 -1; 2 -1; 2 1]  RevolutionCrossSectionUnits=m  RevolutionExtent=Full  RevolutionAngle=180  RevolutionAngleUnits=deg
  World Frame : sm_lib/Frames and Transforms/World Frame
  TH1 : Outport
  TH1_D : Outport  Port=2
  TH1_DD : Outport  Port=3
  TH4 : Outport  Port=4
  TH4_D : Outport  Port=5
  TH4_DD : Outport  Port=6
  wires:
  PS-Simulink Converter/1 -> [TH1]  "TH1"
  PS-Simulink Converter2/1 -> [TH1_DD]  "TH1_DD"
  PS-Simulink Converter1/1 -> [TH1_D]  "TH1_D"
  PS-Simulink Converter9/1 -> [TH4]  "TH4"
  PS-Simulink Converter11/1 -> [TH4_DD]  "TH4_DD"
  PS-Simulink Converter10/1 -> [TH4_D]  "TH4_D"
  TQ_J4/1 -> Simulink-PS Converter/1
  "TQ_J1 "/1 -> Simulink-PS Converter1/1
  [TH1] -> TH1/1
  [TH1_D] -> TH1_D/1
  [TH1_DD] -> TH1_DD/1
  [TH4_DD] -> TH4_DD/1
  [TH4_D] -> TH4_D/1
  [TH4] -> TH4/1
  connections:
  Mechanism Configuration/RConn1 -- RJ_TH4_TURN/LConn1 -- Solver Configuration/RConn1 -- World Frame/RConn1
  Rigid Transform6/LConn1 -- TURNTABLE/RConn1 -- Rigid Transform5/RConn1
  LINK_1/RConn1 -- Rigid Transform/RConn1 -- Rigid Transform1/LConn1
  Simulink-PS Converter1/RConn1 -- RJ_TH1/LConn2
  RZ2LOCY/RConn1 -- Rigid Transform/LConn1
  RJ_TH4_TURN/RConn3 -- PS-Simulink Converter10/LConn1
  PS-Simulink Converter1/LConn1 -- RJ_TH1/RConn3
  LocY2RZ/LConn1 -- Rigid Transform6/RConn1
  Rigid Transform5/LConn1 -- RJ_TH4_TURN/RConn1
  LocY2RZ/RConn1 -- RJ_TH1/LConn1
  LocY2RZ2/LConn1 -- Rigid Transform1/RConn1
  Simulink-PS Converter/RConn1 -- RJ_TH4_TURN/LConn2
  PS-Simulink Converter2/LConn1 -- RJ_TH1/RConn4
  RJ_TH1/RConn1 -- RZ2LOCY/LConn1
  RJ_TH4_TURN/RConn4 -- PS-Simulink Converter11/LConn1
  RJ_TH4_TURN/RConn2 -- PS-Simulink Converter9/LConn1
  PS-Simulink Converter/LConn1 -- RJ_TH1/RConn2

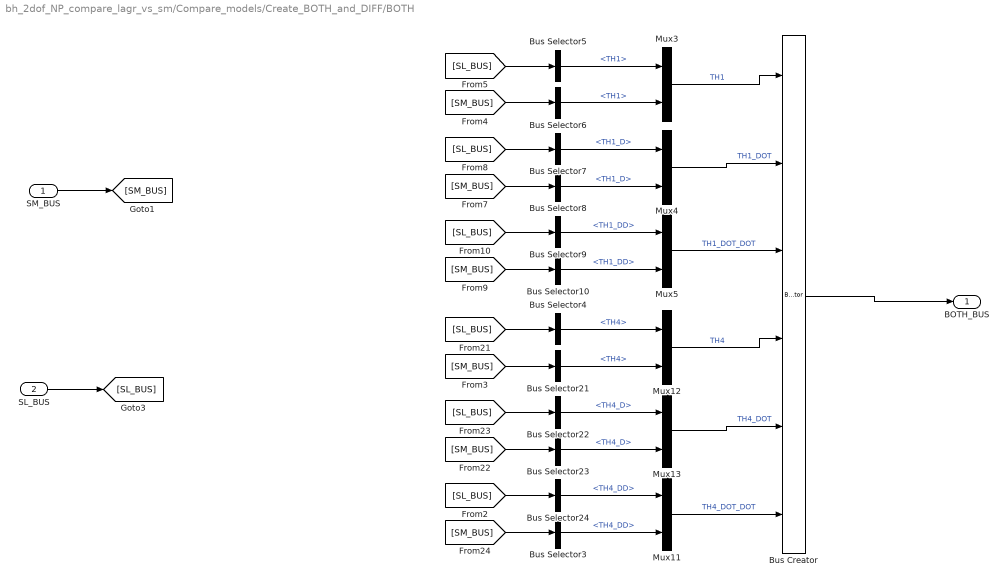
== system bh_2dof_NP_compare_lagr_vs_sm/Compare_models/Create_BOTH_and_DIFF/BOTH ==
  SM_BUS : Inport
  SL_BUS : Inport  Port=2
  Bus Creator : BusCreator  Inputs=6
  Bus Selector10 : BusSelector  OutputSignals=TH1_DD
  Bus Selector21 : BusSelector  OutputSignals=TH4
  Bus Selector22 : BusSelector  OutputSignals=TH4_D
  Bus Selector23 : BusSelector  OutputSignals=TH4_D
  Bus Selector24 : BusSelector  OutputSignals=TH4_DD
  Bus Selector3 : BusSelector  OutputSignals=TH4_DD
  Bus Selector4 : BusSelector  OutputSignals=TH4
  Bus Selector5 : BusSelector  OutputSignals=TH1
  Bus Selector6 : BusSelector  OutputSignals=TH1
  Bus Selector7 : BusSelector  OutputSignals=TH1_D
  Bus Selector8 : BusSelector  OutputSignals=TH1_D
  Bus Selector9 : BusSelector  OutputSignals=TH1_DD
  Mux{3..5,11..13} (6 alike) : Mux  Inputs=2
  BOTH_BUS : Outport
  wires:
  SL_BUS/1 -> [SL_BUS]
  SM_BUS/1 -> [SM_BUS]
  [SM_BUS] -> Bus Selector6/1
  [SL_BUS] -> Bus Selector5/1
  [SL_BUS] -> Bus Selector7/1
  [SM_BUS] -> Bus Selector8/1
  [SL_BUS] -> Bus Selector9/1
  [SM_BUS] -> Bus Selector10/1
  Bus Selector5/1 -> Mux3/1  "<TH1>"
  Bus Selector6/1 -> Mux3/2  "<TH1>"
  Bus Selector7/1 -> Mux4/1  "<TH1_D>"
  Bus Selector8/1 -> Mux4/2  "<TH1_D>"
  Bus Selector9/1 -> Mux5/1  "<TH1_DD>"
  Bus Selector10/1 -> Mux5/2  "<TH1_DD>"
  Mux3/1 -> Bus Creator/1  "TH1"
  Mux4/1 -> Bus Creator/2  "TH1_DOT"
  Bus Creator/1 -> BOTH_BUS/1
  Mux5/1 -> Bus Creator/3  "TH1_DOT_DOT"
  [SM_BUS] -> Bus Selector21/1
  [SL_BUS] -> Bus Selector4/1
  [SL_BUS] -> Bus Selector22/1
  [SM_BUS] -> Bus Selector23/1
  [SL_BUS] -> Bus Selector24/1
  Bus Selector4/1 -> Mux12/1  "<TH4>"
  Bus Selector21/1 -> Mux12/2  "<TH4>"
  Bus Selector22/1 -> Mux13/1  "<TH4_D>"
  Bus Selector23/1 -> Mux13/2  "<TH4_D>"
  Bus Selector24/1 -> Mux11/1  "<TH4_DD>"
  Mux12/1 -> Bus Creator/4  "TH4"
  Mux13/1 -> Bus Creator/5  "TH4_DOT"
  Mux11/1 -> Bus Creator/6  "TH4_DOT_DOT"
  [SM_BUS] -> Bus Selector3/1
  Bus Selector3/1 -> Mux11/2  "<TH4_DD>"

== matlab function bh_2dof_NP_compare_lagr_vs_sm/PLANT_BY_HAND/THE_THETA_SYS_DD ==
  data: L1X_s input; theta1_DD output; L1Y_s input; L1Z_s input; R4_s input; TH1_s input; TH1D_s input; TH4D_s input; b1_s input; b4_s input; g_s input; m1_s input; m4_s input; taum1_s input; taum4_s input; theta4_DD output
function [theta1_DD,theta4_DD] = THE_THETA_SYS_DD(L1X_s,L1Y_s,L1Z_s,R4_s,TH1_s,TH1D_s,TH4D_s,b1_s,b4_s,g_s,m1_s,m4_s,taum1_s,taum4_s)
%#codegen

%    This function was generated by the Symbolic Math Toolbox version 7.2.
%    19-Jul-2017 16:42:27

theta1_DD = (taum1_s.*1.2e1-TH1D_s.*b1_s.*1.2e1-L1Y_s.*g_s.*m1_s.*cos(TH1_s).*6.0-L1Y_s.^2.*TH4D_s.^2.*m1_s.*sin(TH1_s.*2.0).*2.0+L1Z_s.^2.*TH4D_s.^2.*m1_s.*sin(TH1_s.*2.0).*(1.0./2.0))./(L1Y_s.^2.*m1_s.*4.0+L1Z_s.^2.*m1_s);
if nargout > 1
    theta4_DD = (taum4_s.*2.4e1-TH4D_s.*b4_s.*2.4e1+L1Y_s.^2.*TH1D_s.*TH4D_s.*m1_s.*sin(TH1_s.*2.0).*8.0-L1Z_s.^2.*TH1D_s.*TH4D_s.*m1_s.*sin(TH1_s.*2.0).*2.0)./(L1X_s.^2.*m1_s.*2.0+L1Y_s.^2.*m1_s.*4.0+L1Z_s.^2.*m1_s+R4_s.^2.*m4_s.*1.2e1+L1Y_s.^2.*m1_s.*cos(TH1_s.*2.0).*4.0-L1Z_s.^2.*m1_s.*cos(TH1_s.*2.0));
end
